simulink model "BEV_Laengsdynamikmodell_Reiter_1"  (R2022b)
settings: Solver=FixedStepAuto  StartTime=0.0  StopTime=1068  FixedStep=0.001  MaxStep=0.1  RelTol=1e-3  EnableMultiTasking=on
undefined symbols (not defined in the file): gear_ratio, xC, yC, zC
settings Model: Creator=maximilian.tschochne  LastModifiedBy=ga84jar
settings SolverCC: AlgebraicLoopSolver=TrustRegion  AutoInsertRateTranBlk=on
settings DataIOCC: LimitDataPoints=on  SaveFormat=Array  SignalLoggingSaveFormat=ModelDataLogs  ReturnWorkspaceOutputs=off
settings OptimizationCC: BlockReduction=off  OptimizeBlockIOStorage=off  BufferReuse=off  GlobalBufferReuse=off  ExpressionFolding=off  ExpressionDepthLimit=2147483647  LocalBlockOutputs=off  LifeSpan=inf
settings DebuggingCC: UnderspecifiedInitializationDetection=Classic  MergeDetectMultiDrivingBlocksExec=none  SolverPrmCheckMsg=warning  FcnCallInpInsideContextMsg=warning  UnconnectedInputMsg=warning  UnconnectedOutputMsg=warning  UnconnectedLineMsg=warning  StateNameClashWarn=warning  SFUnexpectedBacktrackingDiag=warning  SFNoUnconditionalDefaultTransitionDiag=warning  SFExecutionAtInitializationDiag=none  SFMachineParentedDataDiag=warning  ArithmeticOperatorsInVariantConditions=warning
settings HardwareCC: ProdBitPerPointer=32  ProdBitPerSizeT=32  ProdBitPerPtrDiffT=32  ProdLargestAtomicFloat=None  ProdEndianess=BigEndian  ProdWordSize=32  ProdHWDeviceType=Generic->Custom  TargetIntDivRoundTo=Zero  TargetEndianess=BigEndian  TargetHWDeviceType=Generic->Custom
settings ModelReferenceCC: EnableRefExpFcnMdlSchedulingChecks=on  PropagateSignalLabelsOutOfModel=off
settings SFSimCC: SimUseLocalCustomCode=off  CustomCodeUndefinedFunction=UseInterfaceOnly
settings RTWCC: Description=dSPACE DS1401 Hardware Platform  SystemTargetFile=rti1401.tlc  MakeCommand=make_rti  TemplateMakefile=rti1401.tmf  RTWUseLocalCustomCode=off
settings CodeAppCC: StateflowObjectComments=on
settings STFCustomTargetCC: ParMdlRefBuildCompliant=on  MatFileLogging=on  CPPClassGenCompliant=on  GRTInterface=on  SystemTargetFile=rti1401.tlc
settings GRTTargetCC: TargetLangStandard=C89/C90 (ANSI)  CompOptLevelCompliant=off  ConcurrentExecutionCompliant=off  CombineOutputUpdateFcns=off  GRTInterface=on  UseToolchainInfoCompliant=off  ExtModeMexFile=noextcomm
settings ConfigComp: CovMetricSettings=dw  CovSaveCumulativeToWorkspaceVar=on  CovSaveSingleToWorkspaceVar=on  CovExternalEMLEnable=off  CovSFcnEnable=off  DVTestSuiteOptimization=Auto  DVDetectOutOfBounds=on  DVModelReferenceHarness=on  DVHarnessSource=Signal Editor

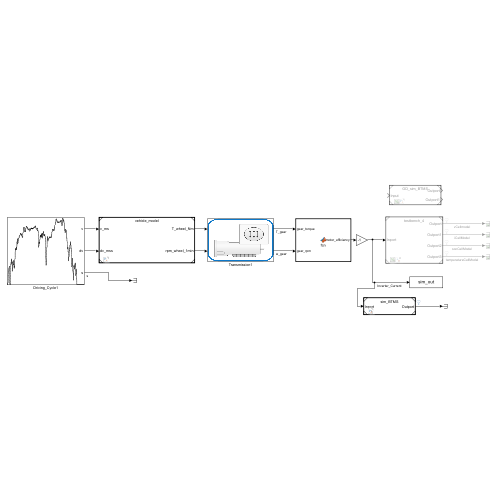
[thumbnail: Simulink's stored preview of the top-level diagram]
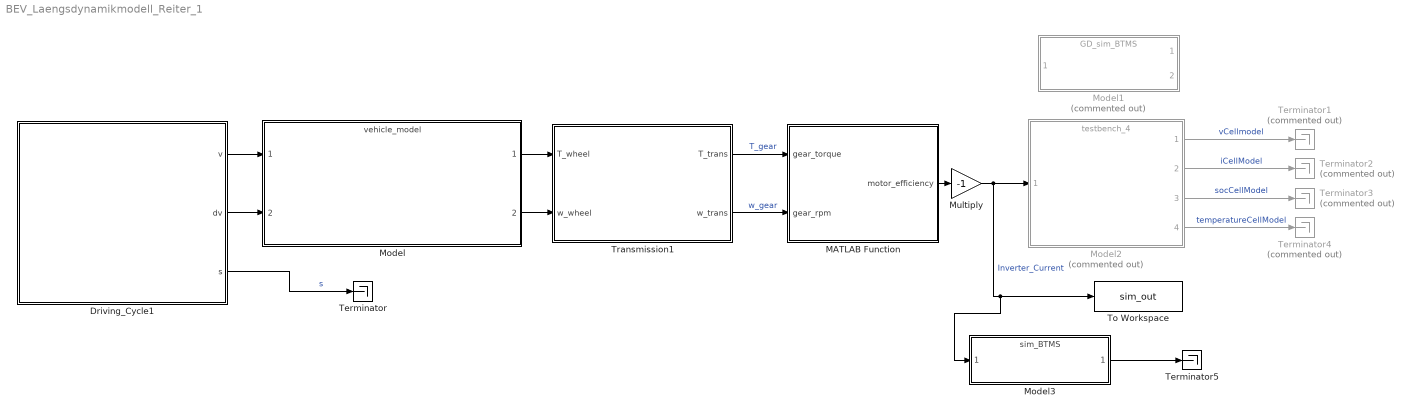
== system BEV_Laengsdynamikmodell_Reiter_1 ==
  Driving_Cycle1 : Subsystem  mask{dcname=EUROPE_ARTEMIS_MOTORWAY, ShowDCPlot=off}
      mask prompts: dcname "Choose Driving Cycle"; ShowDCPlot "Show DC Plot"
      mask init:
      | init_driving_cycle
      mask TypeOptions dcname: EUROPE_ARTEMIS_MOTORWAY | EUROPE_ARTEMIS_ROAD | EUROPE_ARTEMIS_URBAN | EUROPE_City | EUROPE_EUDC | EUROPE_NEDC | EUROPE_UDC | JAPAN_10_15_MODE | JAPAN_10_MODE | JAPAN_10_MODE_3 | JAPAN_11_MODE | JAPAN_11_MODE_4 | JAPAN_15_MODE | USA_CITY_I | USA_CITY_II | USA_FTP_72 | USA_FTP_75 | USA_FTP_HIGHWAY | USA_NECC | WLTP_class_3
      mask Display:
      | port_label('output',1,'v');
      | port_label('output',2,'dv');
      | port_label('output',3,'s');
      | plot(T_zplot, V_zplot);
  MATLAB Function : MATLAB Function  TreatAsAtomicUnit=on
  Model : ModelReference  ModelNameDialog=vehicle_model.slx  SimulationMode=Normal  ModelReferenceVersion=1.13
  Model1 : ModelReference  Commented=on  ModelNameDialog=GD_sim_BTMS.slx  SimulationMode=Normal  ModelReferenceVersion=5.2
  Model2 : ModelReference  Commented=on  ModelNameDialog=testbench_4.slx  SimulationMode=Normal  ModelReferenceVersion=1.17
  Model3 : ModelReference  ModelNameDialog=sim_BTMS.slx  SimulationMode=Normal  ModelReferenceVersion=5.1
  Multiply : Gain  Gain=-1
  Terminator : Terminator
  Terminator{1..4} (4 alike) : Terminator  Commented=on
  Terminator5 : Terminator
  To Workspace : ToWorkspace  VariableName=sim_out  SampleTime=-1
  Transmission1 : Subsystem  mask{i=gear_ratio, eta=0.95}
      mask prompts: i "Transmission Ratio"; eta "Tranmisstion Efficiency"
      mask Display: image('Transmission.png')
  wires:
  Driving_Cycle1/1(v) -> Model/1
  Driving_Cycle1/2(dv) -> Model/2
  Model/1 -> Transmission1/1(T_wheel)
  Transmission1/1(T_trans) -> MATLAB Function/1(gear_torque)  "T_gear"
  Transmission1/2(w_trans) -> MATLAB Function/2(gear_rpm)  "w_gear"
  Model/2 -> Transmission1/2(w_wheel)
  Multiply/1 -> Model2/1, Model3/1, To Workspace/1  "Inverter_Current"
  Driving_Cycle1/3(s) -> Terminator/1  "s"
  Model2/1 -> Terminator1/1  "vCellmodel"
  Model2/2 -> Terminator2/1  "iCellModel"
  Model2/3 -> Terminator3/1  "socCellModel"
  Model2/4 -> Terminator4/1  "temperatureCellModel"
  MATLAB Function/1(motor_efficiency) -> Multiply/1
  Model3/1 -> Terminator5/1

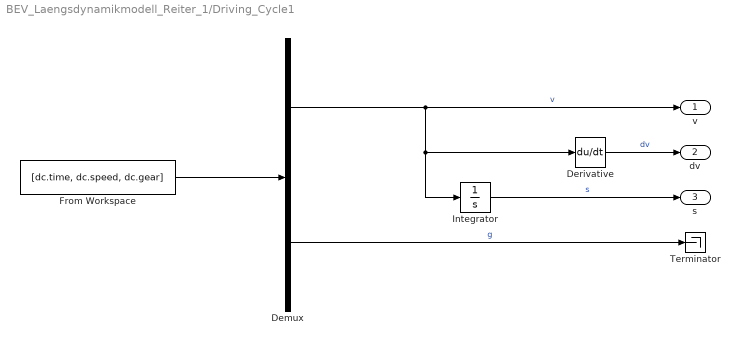
== system BEV_Laengsdynamikmodell_Reiter_1/Driving_Cycle1 ==
  Demux : Demux  Outputs=2
  Derivative : Derivative
  From Workspace : FromWorkspace  VariableName=[dc.time, dc.speed, dc.gear]
  Integrator : Integrator
  Terminator : Terminator
  v : Outport  VectorParamsAs1DForOutWhenUnconnected=off
  dv : Outport  Port=2  VectorParamsAs1DForOutWhenUnconnected=off
  s : Outport  Port=3  VectorParamsAs1DForOutWhenUnconnected=off
  wires:
  Integrator/1 -> s/1  "s"
  Demux/2 -> Terminator/1  "g"
  Derivative/1 -> dv/1  "dv"
  From Workspace/1 -> Demux/1
  Demux/1 -> v/1, Integrator/1, Derivative/1  "v"

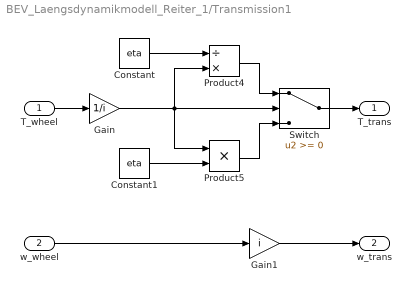
== system BEV_Laengsdynamikmodell_Reiter_1/Transmission1 ==
  T_wheel : Inport
  w_wheel : Inport  Port=2
  Constant : Constant  Value=eta
  Constant1 : Constant  Value=eta
  Gain : Gain  Gain=1/i
  Gain1 : Gain  Gain=i
  Product4 : Product  Inputs=/*  RndMeth=Zero
  Product5 : Product  RndMeth=Zero
  Switch : Switch  SaturateOnIntegerOverflow=off  InputSameDT=off
  T_trans : Outport  VectorParamsAs1DForOutWhenUnconnected=off
  w_trans : Outport  Port=2  VectorParamsAs1DForOutWhenUnconnected=off
  wires:
  T_wheel/1 -> Gain/1
  w_wheel/1 -> Gain1/1
  Gain1/1 -> w_trans/1
  Switch/1 -> T_trans/1
  Product4/1 -> Switch/1
  Product5/1 -> Switch/3
  Constant/1 -> Product4/1
  Constant1/1 -> Product5/2
  Gain/1 -> Switch/2, Product4/2, Product5/1

== matlab function BEV_Laengsdynamikmodell_Reiter_1/MATLAB Function ==
  data: gear_torque input; motor_efficiency output; gear_rpm input; xC parameter; yC parameter; zC parameter
function motor_efficiency = fcn(gear_torque, gear_rpm, xC, yC, zC)
    % this function calculates the efficency/current of the motor and electronics
    % from an efficiency map including motor torque and speed.

    diff_mat = zeros(1, size(xC, 2));
    for idx = 1:size(xC, 2)
        diff_mat(idx) = min(abs(xC{idx}-gear_rpm) + abs(yC{idx}-gear_torque));
    end
    [~, idx_min] = min(diff_mat);
    motor_efficiency = zC{idx_min};
    motor_efficiency = sign(gear_torque) * motor_efficiency;
